simulink model "Lab03_Q3_Sim"  (R2024a)
settings: Solver=VariableStepAuto  StartTime=0.0  StopTime=600  RelTol=1e-3
values from neighbouring files (symbols this model uses):
  C_T = H'    [Lab03_Q3.m]    (also in Lab03_Q3_Data.mat = [0 1])
  DC_gain3 = 1 / gain_ndb3    [Lab03_Q3.m]    (also in Lab03_Q3_Data.mat = 0.270995247235)
  G_T = G'    [Lab03_Q3.m]    (also in Lab03_Q3_Data.mat = [0  -0.559342138353; 1  1.54391351652])
  h = t(2) - t(1)    [Lab03_Q3.m]
  H_T = C'    [Lab03_Q3.m]    (also in Lab03_Q3_Data.mat = [0.0106247741063 0.0262762420629])
  K_db = (acker(G, H, [0 0]))'    [Lab03_Q3.m]    (also in Lab03_Q3_Data.mat = [-0.559342138353 1.54391351652])
  L_ndb3 = acker(G_T, H_T, [0.9 0.9])    [Lab03_Q3.m]    (also in Lab03_Q3_Data.mat = [-10.0065993924 -5.69977339244])
libraries: simulink x1
settings Model: Creator=24246  LastModifiedBy=24246
settings DataIOCC: ReturnWorkspaceOutputs=off

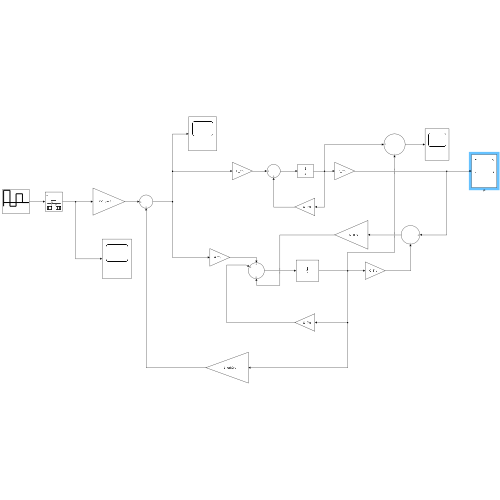
[thumbnail: Simulink's stored preview of the top-level diagram]
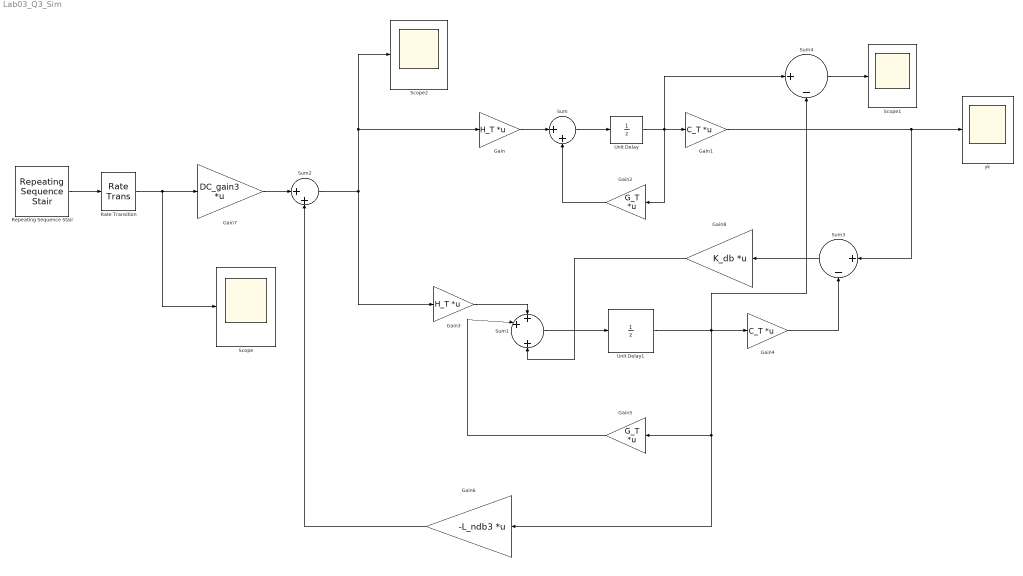
== system Lab03_Q3_Sim ==
  Gain : Gain  Gain=H_T  Multiplication=Matrix(K*u)
  Gain1 : Gain  Gain=C_T  Multiplication=Matrix(K*u)
  Gain2 : Gain  Gain=G_T  Multiplication=Matrix(K*u)
  Gain3 : Gain  Gain=H_T  Multiplication=Matrix(K*u)
  Gain4 : Gain  Gain=C_T  Multiplication=Matrix(K*u)
  Gain5 : Gain  Gain=G_T  Multiplication=Matrix(K*u)
  Gain6 : Gain  Gain=-L_ndb3  Multiplication=Matrix(K*u)
  Gain7 : Gain  Gain=DC_gain3  Multiplication=Matrix(K*u)
  Gain8 : Gain  Gain=K_db  Multiplication=Matrix(K*u)
  Rate Transition : RateTransition  OutPortSampleTime=h
  Repeating Sequence Stair : simulink/Sources/Repeating Sequence Stair  OutValues=[0.7 -0.2 0.5 0]'  tsamp=105  OutMin=[]  OutMax=[]  OutDataTypeStr=double  OutputDataTypeScalingMode=double  OutDataType=fixdt(0,8)  ConRadixGroup=Best Precision: Vector-wise  OutScaling=2^-12
  Scope : Scope
  Scope1 : Scope
  Scope2 : Scope
  Sum : Sum  Inputs=|++
  Sum1 : Sum  Inputs=++|+
  Sum2 : Sum  Inputs=|++
  Sum3 : Sum  Inputs=|+-
  Sum4 : Sum  Inputs=|+-
  Unit Delay : UnitDelay  InitialCondition=[0 0]  SampleTime=h  HasFrameUpgradeWarning=on
  Unit Delay1 : UnitDelay  InitialCondition=[0 0]  SampleTime=h  HasFrameUpgradeWarning=on
  yk : Scope
  wires:
  Gain/1 -> Sum/1
  Sum/1 -> Unit Delay/1
  Unit Delay/1 -> Sum4/1, Gain2/1, Gain1/1
  Gain2/1 -> Sum/2
  Gain3/1 -> Sum1/1
  Unit Delay1/1 -> Sum4/2, Gain4/1, Gain6/1, Gain5/1
  Sum2/1 -> Gain3/1, Scope2/1, Gain/1
  Gain6/1 -> Sum2/2
  Gain7/1 -> Sum2/1
  Gain5/1 -> Sum1/2
  Gain8/1 -> Sum1/3
  Sum1/1 -> Unit Delay1/1
  Sum3/1 -> Gain8/1
  Gain4/1 -> Sum3/2
  Gain1/1 -> Sum3/1, yk/1
  Repeating Sequence Stair/1 -> Rate Transition/1
  Rate Transition/1 -> Scope/1, Gain7/1
  Sum4/1 -> Scope1/1
